simulink model "SRG_Generic_1HpSepExt_13Jan15_mod1"  (Simulink 8.1)
settings: Solver=ode45  StartTime=0.0  StopTime=2.5  FixedStep=Ts  MaxStep=1e-6  MinStep=1e-7  RelTol=1e-5
values from neighbouring files (symbols this model uses):
  Ts = 1e-06    [WorkSpaceBackup1.mat]
undefined symbols (not defined in the file or in its folder): DiscIntNeverNeededParam, find_system
libraries: powerlib x29, simulink x2, powerlib_extras x2, dspsigops x1, DRlib x1
settings Model: Creator=Rahul  LastModifiedBy=USER
settings DataIOCC: SignalLoggingName=signout
settings OptimizationCC: InitFltsAndDblsToZero=on
settings DebuggingCC: CheckExecutionContextPreStartOutputMsg=on  CheckExecutionContextRuntimeOutputMsg=on  SolverPrmCheckMsg=none  MultiTaskDSMMsg=warning  MultiTaskCondExecSysMsg=none
settings HardwareCC: TargetHWDeviceType=32-bit Generic

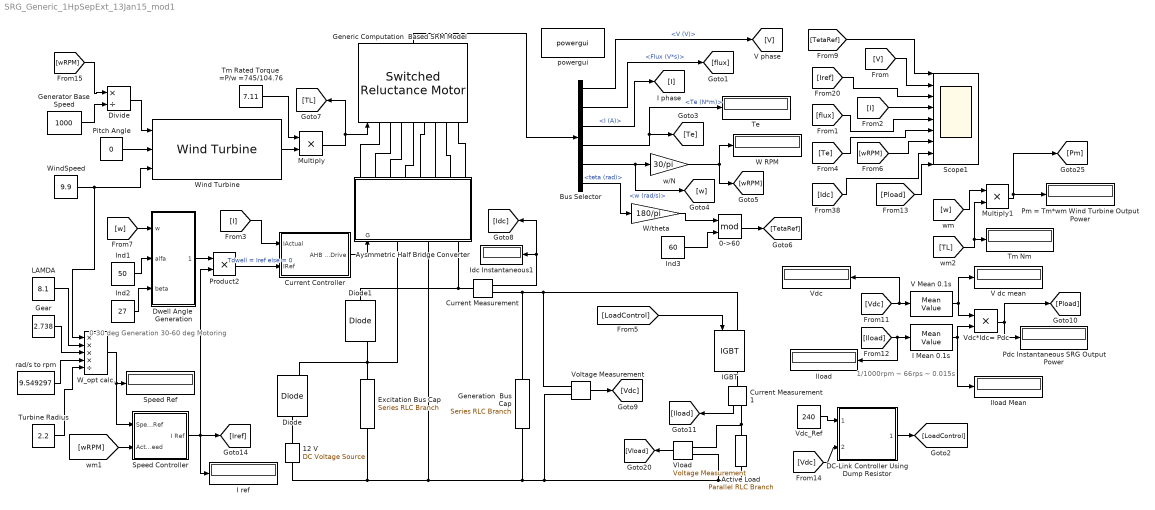
== system SRG_Generic_1HpSepExt_13Jan15_mod1 ==
  note: 1/1000rpm ~ 66rps ~ 0.015s
  note: 0-30 deg Generation
      | 30-60 deg Motoring
  0->60 : Math  Operator=mod  SampleTime=Ts  SaturateOnIntegerOverflow=on
  12 V : powerlib/Electrical Sources/DC Voltage Source  Amplitude=12  Measurements=None
  Active Load : powerlib/Elements/Parallel RLC Branch  LConnTagsString=a  RConnTagsString=__new0  BranchType=R  Resistance=1  Inductance=1e-3  SetiL0=off  InitialCurrent=0  Capacitance=1e-6  Setx0=off  InitialVoltage=0  Measurements=None
  Aysmmetric Half Bridge Converter : Subsystem  LoadFcn=find_system(gcs,'FollowLinks', 'on', 'LookUnderMasks', 'all');
  Bus Selector : BusSelector  OutputSignals=V (V),Flux (V*s),I (A),Te (N*m),w (rad/s),teta (rad)
  Current Controller : Subsystem
  Current Measurement : powerlib/Measurements/Current Measurement  PhasorSimulation=off  OutputType=Complex  PSBequivalent=0
  Current Measurement1 : powerlib/Measurements/Current Measurement  PhasorSimulation=off  OutputType=Complex  PSBequivalent=0
  "DC-Link Controller Using Dump Resistor " : Subsystem
  Diode : powerlib/Power Electronics/Diode  Ron=0.001  Lon=0  Vf=0.8  IC=0  UseSnubber=off  Rs=10e6  Cs=inf  Measurements=on
  Diode1 : powerlib/Power Electronics/Diode  Ron=0.001  Lon=0  Vf=0.8  IC=0  UseSnubber=off  Rs=10e6  Cs=inf  Measurements=on
  Divide : Product  Inputs=*/
  Dwell Angle  Generation : Subsystem
  Excitation Bus Cap : powerlib/Elements/Series RLC Branch  LConnTagsString=__new0  RConnTagsString=__new0  BranchType=RC  Resistance=0.001  Inductance=1e-3  SetiL0=off  InitialCurrent=0  Capacitance=3000e-6  Setx0=on  InitialVoltage=1  Measurements=None
  Gear : Constant  Value=2.738
  Generation  Bus Cap : powerlib/Elements/Series RLC Branch  LConnTagsString=__new0  RConnTagsString=__new0  BranchType=RC  Resistance=0.001  Inductance=1e-3  SetiL0=off  InitialCurrent=0  Capacitance=3000e-6  Setx0=on  InitialVoltage=1  Measurements=None
  Generator Base Speed : Constant  Value=1000
  "Generic Computation  Based SRM Model  " : powerlib/Machines/Switched Reluctance Motor  MachineType=8/6  MachineModel=Generic model  StatorResistance=0.013  PlotCurves=off  Inertia=0.004  Friction=0  InitialSpeed=[97 0]  Lq=0.008  Ld=0.32  Lsat=0.0005  MaximumCurrent=6  MaximumFluxLinkage=0.4  MagnetisationCharacteristic='srm64_60kw.mat'  RotorAngleVector=[0 10 20 30 40 45]  StatorCurrentVector=0:25:450  TsPowergui=0  TsBlock=-1
  I Mean 0.1s : powerlib_extras/Measurements/Mean Value  Period=0.015
  I ref : Display
  IGBT : powerlib/Power Electronics/IGBT  Ron=0.001  Lon=0  Vf=1  Tf=1e-6  Tt=2e-6  IC=0  Rs=1e5  Cs=inf  Measurements=on
  Idc Instantaneous1 : Display
  "Iload " : Display
  Iload Mean : Display
  Ind1 : Constant  Value=50
  Ind2 : Constant  Value=27
  Ind3 : Constant  Value=60
  LAMDA : Constant  Value=8.1
  Multiply : Product  Inputs=**
  Multiply1 : Product  Inputs=**
  Pdc Instantaneous SRG Output Power : Display
  Pitch Angle : Constant  Value=0
  Pm = Tm*wm Wind Turbine Output Power : Display
  Product2 : Product  RndMeth=Zero
  Scope1 : Scope  NumInputPorts=9
      settings: TimeRange=0.1400000000000001  YMin=0~-300~0~-2~-0.1~-10~900~-250~0  YMax=100~300~12~10~0.5~5~1500~250~800  SaveName=ScopeData2  MaxDataPoints=100000
  Speed Controller : Subsystem
  Speed Ref : Display
  Te : Display
  Tm Nm : Display
  Tm Rated Torque =P/w =745/104.76 : Constant  Value=7.11
  Turbine Radius : Constant  Value=2.2
  V Mean 0.1s : powerlib_extras/Measurements/Mean Value  Period=0.015
  V dc mean : Display
  "Vdc " : Display
  Vdc*Idc= Pdc : Product
  Vdc_Ref : Constant  Value=240
  Vload : powerlib/Measurements/Voltage Measurement  PhasorSimulation=off  OutputType=Complex  PSBequivalent=0
  Voltage Measurement : powerlib/Measurements/Voltage Measurement  PhasorSimulation=off  OutputType=Complex  PSBequivalent=0
  W RPM : Display
  W/theta : Gain  Gain=180/pi
  W_opt calc. : Product  Inputs=****/
  Wind Turbine : DRlib/Wind Generation/Wind Turbine  Pnom=1e3  Pelec_base=1e3/0.9  wind_base=12.5  P_wind_base=1  speed_nom=1.2  pitch_angle=0  DisplayTurbChar=off  c1_c6="[0.51763          116          0.4            5           21     0.006795]"  cp_nom=0.48  lambda_nom=8.1
  WindSpeed : Constant  Value=9.9
  powergui : powerlib/powergui  Priority=1  SimulationMode=Discrete  SolverType=Tustin  SampleTime=Ts  frequency=60  SPID=off  DisableSnubberDevices=off  DisableRonSwitches=off  DisableVfSwitches=off  SwTol=0  Interpol=off  DisplayEquations=off  frequencyindice=0  Pbase=100e6  ErrMax=1e-4  Iterations=50  UnitsV=kV  UnitsW=MW  FunctionMessages=off  echomessages=off  HookPort=off  EnableUseOfTLC=off  x0status=blocks  RestoreLinks=warning  ResistiveCurrentMeasurement=off  Frange=[0:2:500]  Ylog=off  Xlog=on  ShowGrid=off  save=off  variable=ZData  ZoomFFT=off  StartTime=0.0  cycles=1  DisplayStyle=1  fundamental=60  FreqAxis=off  MaxFrequency=1000  frequencyindicesteady=1  RmsSteady=1  display=off  Ts=0  methode=off
  rad/s to rpm : Constant  Value=9.549297
  w/N : Gain  Gain=30/pi
  wires:
  "Generic Computation  Based SRM Model  "/1 -> Bus Selector/1
  Bus Selector/6 -> W/theta/1  "<teta (rad)>"
  w/N/1 -> [wRPM], W RPM/1
  Ind3/1 -> 0->60/2
  W/theta/1 -> 0->60/1
  Bus Selector/1 -> [V]  "<V (V)>"
  Bus Selector/2 -> [flux]  "<Flux (V*s)>"
  Bus Selector/3 -> [I]  "<I (A)>"
  Bus Selector/4 -> [Te], Te/1  "<Te (N*m)>"
  Bus Selector/5 -> w/N/1, [w]  "<w (rad/s)>"
  0->60/1 -> [TetaRef]
  Voltage Measurement/1 -> [Vdc]
  Current Measurement/1 -> Idc Instantaneous1/1, [Idc]
  [Iload] -> "Iload "/1, I Mean 0.1s/1
  Vdc*Idc= Pdc/1 -> Pdc Instantaneous SRG Output Power/1, [Pload]
  Current Measurement1/1 -> [Iload]
  [w] -> Multiply1/1
  Multiply1/1 -> [Pm], Pm = Tm*wm Wind Turbine Output Power/1
  [Vdc] -> "Vdc "/1, V Mean 0.1s/1
  I Mean 0.1s/1 -> Iload Mean/1, Vdc*Idc= Pdc/2
  Vload/1 -> [Vload]
  V Mean 0.1s/1 -> V dc mean/1, Vdc*Idc= Pdc/1
  Ind1/1 -> Dwell Angle  Generation/2(alfa)
  Ind2/1 -> Dwell Angle  Generation/3(beta)
  [w] -> Dwell Angle  Generation/1(w)
  [TetaRef] -> Scope1/1
  [V] -> Scope1/2
  [Iref] -> Scope1/3
  [I] -> Scope1/4
  [Pload] -> Scope1/9
  [Idc] -> Scope1/8
  [wRPM] -> Scope1/7
  [Te] -> Scope1/6
  [flux] -> Scope1/5
  [LoadControl] -> IGBT/1
  Vdc_Ref/1 -> "DC-Link Controller Using Dump Resistor "/1(Ref Gen Bus V)
  [Vdc] -> "DC-Link Controller Using Dump Resistor "/2(Actual Gen Bus V)
  "DC-Link Controller Using Dump Resistor "/1(" Load Gate") -> [LoadControl]
  Speed Controller/1(I Ref) -> I ref/1, [Iref], Product2/2
  [wRPM] -> Speed Controller/2(ActualSpeed)
  Product2/1 -> Current Controller/2(IRef)  "Tdwell = Iref else = 0"
  [I] -> Current Controller/1(IActual)
  Current Controller/1(AHB GateDrive) -> Aysmmetric Half Bridge Converter/1(G)
  Dwell Angle  Generation/1(Signal) -> Product2/1
  [wRPM] -> Divide/1
  Generator Base Speed/1 -> Divide/2
  Divide/1 -> Wind Turbine/1
  Pitch Angle/1 -> Wind Turbine/2
  WindSpeed/1 -> W_opt calc./1, Wind Turbine/3
  Multiply/1 -> [TL], "Generic Computation  Based SRM Model  "/1
  Wind Turbine/1 -> Multiply/2
  Tm Rated Torque =P/w =745/104.76/1 -> Multiply/1
  [TL] -> Multiply1/2, Tm Nm/1
  Gear/1 -> W_opt calc./3
  LAMDA/1 -> W_opt calc./2
  Turbine Radius/1 -> W_opt calc./5
  rad/s to rpm/1 -> W_opt calc./4
  W_opt calc./1 -> Speed Ref/1, Speed Controller/1(SpeedRef)
  connections:
  "Generic Computation  Based SRM Model  "/LConn1 -- Aysmmetric Half Bridge Converter/RConn1
  "Generic Computation  Based SRM Model  "/LConn2 -- Aysmmetric Half Bridge Converter/RConn2
  "Generic Computation  Based SRM Model  "/LConn3 -- Aysmmetric Half Bridge Converter/RConn3
  "Generic Computation  Based SRM Model  "/LConn4 -- Aysmmetric Half Bridge Converter/RConn4
  "Generic Computation  Based SRM Model  "/LConn5 -- Aysmmetric Half Bridge Converter/RConn5
  "Generic Computation  Based SRM Model  "/LConn6 -- Aysmmetric Half Bridge Converter/RConn6
  Voltage Measurement/LConn2 -- Active Load/RConn1 -- Vload/LConn2 -- Generation  Bus Cap/RConn1 -- 12 V/LConn1 -- Excitation Bus Cap/RConn1 -- Aysmmetric Half Bridge Converter/LConn2
  Voltage Measurement/LConn1 -- IGBT/LConn1 -- Current Measurement/RConn1 -- Generation  Bus Cap/LConn1
  Diode/LConn1 -- 12 V/RConn1
  Active Load/LConn1 -- Vload/LConn1 -- Current Measurement1/RConn1
  IGBT/RConn1 -- Current Measurement1/LConn1
  Aysmmetric Half Bridge Converter/RConn7 -- "Generic Computation  Based SRM Model  "/LConn7
  Aysmmetric Half Bridge Converter/RConn8 -- "Generic Computation  Based SRM Model  "/LConn8
  Aysmmetric Half Bridge Converter/LConn3 -- Current Measurement/LConn1 -- Diode1/LConn1
  Aysmmetric Half Bridge Converter/LConn1 -- Diode/RConn1 -- Excitation Bus Cap/LConn1 -- Diode1/RConn1

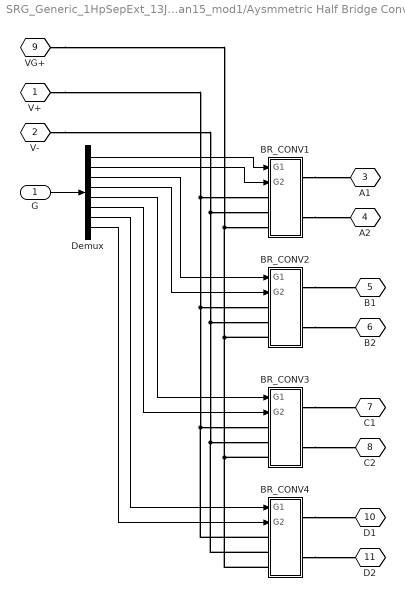
== system SRG_Generic_1HpSepExt_13Jan15_mod1/Aysmmetric Half Bridge Converter ==
  G : Inport
  BR_CONV1 : Subsystem
  BR_CONV2 : Subsystem
  BR_CONV3 : Subsystem
  BR_CONV4 : Subsystem
  Demux : Demux  Outputs=8
  V+ : PMIOPort  Tag=PMCPort  Port=1  Side=Left
  V- : PMIOPort  Tag=PMCPort  Port=2  Side=Left
  A1 : PMIOPort  Tag=PMCPort  Port=3  Side=Right
  A2 : PMIOPort  Tag=PMCPort  Port=4  Side=Right
  B1 : PMIOPort  Tag=PMCPort  Port=5  Side=Right
  B2 : PMIOPort  Tag=PMCPort  Port=6  Side=Right
  C1 : PMIOPort  Tag=PMCPort  Port=7  Side=Right
  C2 : PMIOPort  Tag=PMCPort  Port=8  Side=Right
  VG+ : PMIOPort  Tag=PMCPort  Port=9  Side=Left
  D1 : PMIOPort  Tag=PMCPort  Port=10  Side=Right
  D2 : PMIOPort  Tag=PMCPort  Port=11  Side=Right
  wires:
  G/1 -> Demux/1
  Demux/1 -> BR_CONV1/1(G1)
  Demux/2 -> BR_CONV1/2(G2)
  Demux/3 -> BR_CONV2/1(G1)
  Demux/4 -> BR_CONV2/2(G2)
  Demux/5 -> BR_CONV3/1(G1)
  Demux/6 -> BR_CONV3/2(G2)
  Demux/7 -> BR_CONV4/1(G1)
  Demux/8 -> BR_CONV4/2(G2)
  connections:
  BR_CONV3/RConn2 -- C2/RConn1
  BR_CONV3/RConn1 -- C1/RConn1
  BR_CONV2/RConn2 -- B2/RConn1
  BR_CONV2/RConn1 -- B1/RConn1
  BR_CONV1/RConn2 -- A2/RConn1
  BR_CONV1/RConn1 -- A1/RConn1
  V-/RConn1 -- BR_CONV1/LConn2 -- BR_CONV4/LConn2 -- BR_CONV3/LConn2 -- BR_CONV2/LConn2
  V+/RConn1 -- BR_CONV1/LConn1 -- BR_CONV4/LConn1 -- BR_CONV3/LConn1 -- BR_CONV2/LConn1
  VG+/RConn1 -- BR_CONV1/LConn3 -- BR_CONV4/LConn3 -- BR_CONV3/LConn3 -- BR_CONV2/LConn3
  BR_CONV4/RConn2 -- D2/RConn1
  BR_CONV4/RConn1 -- D1/RConn1

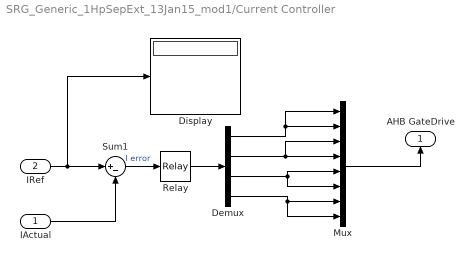
== system SRG_Generic_1HpSepExt_13Jan15_mod1/Current Controller ==
  IActual : Inport
  IRef : Inport  Port=2
  Demux : Demux
  Display : Display
  Mux : Mux  Inputs=8
  Relay : Relay  OnSwitchValue=0.1  OffSwitchValue=-0.1
  Sum1 : Sum  Inputs=|+-
  AHB GateDrive : Outport
  wires:
  IRef/1 -> Display/1, Sum1/1
  Sum1/1 -> Relay/1  "I error"
  IActual/1 -> Sum1/2
  Relay/1 -> Demux/1
  Demux/1 -> Mux/1, Mux/2
  Demux/2 -> Mux/3, Mux/4
  Demux/3 -> Mux/6, Mux/5
  Demux/4 -> Mux/8, Mux/7
  Mux/1 -> AHB GateDrive/1

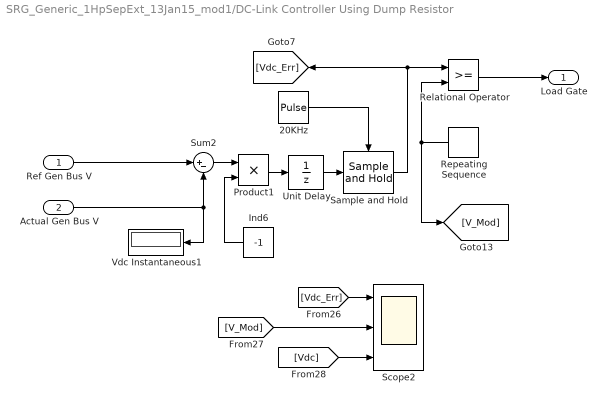
== system SRG_Generic_1HpSepExt_13Jan15_mod1/DC-Link Controller Using Dump Resistor  ==
  Ref Gen Bus V : Inport
  Actual Gen Bus V : Inport  Port=2
  20KHz : DiscretePulseGenerator  PulseType=Time based  Period=0.5e-4  PulseWidth=10
  Ind6 : Constant  Value=-1
  Product1 : Product
  Relational Operator : RelationalOperator  OutDataTypeStr=boolean
  Repeating Sequence : simulink/Sources/Repeating Sequence  rep_seq_t=[0 0.25e-4 0.5e-4]  rep_seq_y=[0 1 0]
  Sample and Hold : dspsigops/Sample and Hold  trig=Rising edge  initCond=0  latchinput=off
  Scope2 : Scope  NumInputPorts=3
      settings: TimeRange=0.1400000000000001  YMin=-5~-2~0  YMax=5~2~300  MaxDataPoints=100000
  Sum2 : Sum  Inputs=|+-
  Unit Delay : UnitDelay  SampleTime=-1
  Vdc Instantaneous1 : Display
  " Load Gate" : Outport
  wires:
  Ref Gen Bus V/1 -> Sum2/1
  Actual Gen Bus V/1 -> Sum2/2, Vdc Instantaneous1/1
  [V_Mod] -> Scope2/2
  [Vdc] -> Scope2/3
  20KHz/1 -> Sample and Hold/Trigger
  Repeating Sequence/1 -> Relational Operator/2, [V_Mod]
  [Vdc_Err] -> Scope2/1
  Ind6/1 -> Product1/2
  Product1/1 -> Unit Delay/1
  Unit Delay/1 -> Sample and Hold/1
  Sample and Hold/1 -> Relational Operator/1, [Vdc_Err]
  Sum2/1 -> Product1/1
  Relational Operator/1 -> " Load Gate"/1

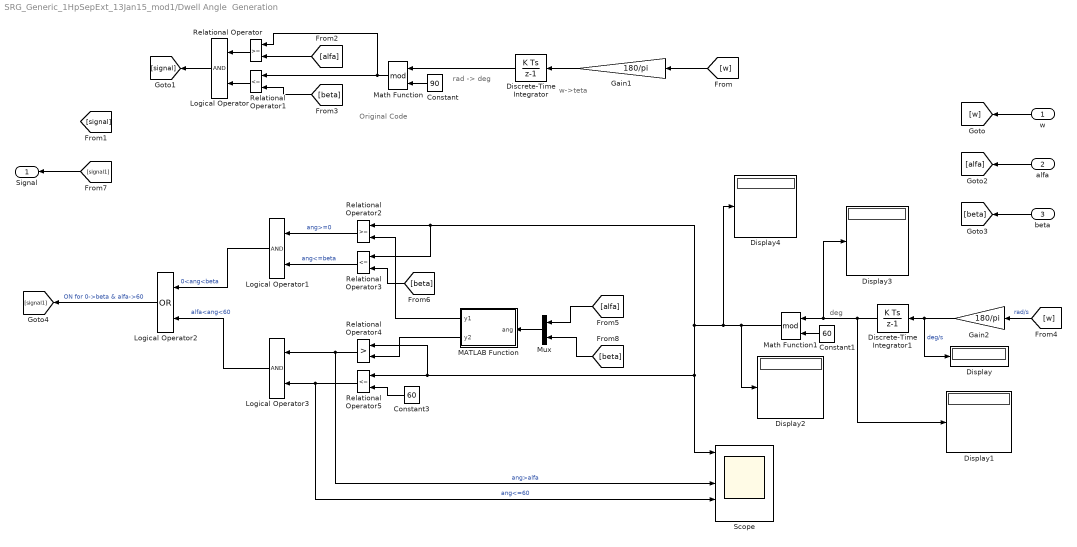
== system SRG_Generic_1HpSepExt_13Jan15_mod1/Dwell Angle  Generation ==
  note: Original Code
  note: rad -> deg
  note: w->teta
  note: deg
  w : Inport
  alfa : Inport  Port=2
  beta : Inport  Port=3
  Constant : Constant  Value=90
  Constant1 : Constant  Value=60
  Constant3 : Constant  Value=60
  Discrete-Time Integrator : DiscreteIntegrator  InitialCondition=[0 -30 -60]  SampleTime=Ts  ICPrevOutput=DiscIntNeverNeededParam  ICPrevScaledInput=DiscIntNeverNeededParam
  Discrete-Time Integrator1 : DiscreteIntegrator  InitialCondition=[0 -15 -30 -45]  SampleTime=Ts  ICPrevOutput=DiscIntNeverNeededParam  ICPrevScaledInput=DiscIntNeverNeededParam
  Display{,1..4} (5 alike) : Display
  Gain1 : Gain  Gain=180/pi  SaturateOnIntegerOverflow=on  OutDataTypeStr=Inherit: Same as input  ParamDataTypeStr=Inherit: Same as input
  Gain2 : Gain  Gain=180/pi  SaturateOnIntegerOverflow=on  OutDataTypeStr=Inherit: Same as input  ParamDataTypeStr=Inherit: Same as input
  Logical Operator : Logic  AllPortsSameDT=off
  Logical Operator1 : Logic  AllPortsSameDT=off
  Logical Operator2 : Logic  Operator=OR  AllPortsSameDT=off
  Logical Operator3 : Logic  AllPortsSameDT=off
  MATLAB Function : MATLAB Function  TreatAsAtomicUnit=on
  Math Function : Math  Operator=mod  SaturateOnIntegerOverflow=on
  Math Function1 : Math  Operator=mod  SaturateOnIntegerOverflow=on
  Mux : Mux  Inputs=2
  Relational Operator : RelationalOperator
  Relational Operator1 : RelationalOperator  Operator=<=
  Relational Operator2 : RelationalOperator
  Relational Operator3 : RelationalOperator  Operator=<=
  Relational Operator4 : RelationalOperator  Operator=>
  Relational Operator5 : RelationalOperator  Operator=<=
  Scope : Scope  NumInputPorts=5
      settings: YMin=-5~-5~-5~-5~-5  YMax=5~5~5~5~5
  Signal : Outport
  wires:
  Math Function/1 -> Relational Operator/1, Relational Operator1/1
  Relational Operator1/1 -> Logical Operator/2
  beta/1 -> [beta]
  alfa/1 -> [alfa]
  Relational Operator/1 -> Logical Operator/1
  Constant/1 -> Math Function/2
  Logical Operator/1 -> [signal]
  Discrete-Time Integrator/1 -> Math Function/1
  Gain1/1 -> Discrete-Time Integrator/1
  w/1 -> [w]
  [w] -> Gain2/1  "rad/s"
  Math Function1/1 -> Display2/1, Relational Operator3/1, Relational Operator2/1, Scope/1, Relational Operator4/1, Relational Operator5/1, Display4/1
  Gain2/1 -> Display/1, Discrete-Time Integrator1/1  "deg/s"
  [beta] -> Relational Operator3/2
  Relational Operator2/1 -> Logical Operator1/1  "ang>=0"
  Constant1/1 -> Math Function1/2
  Discrete-Time Integrator1/1 -> Display1/1, Math Function1/1, Display3/1
  Relational Operator3/1 -> Logical Operator1/2  "ang<=beta"
  Logical Operator1/1 -> Logical Operator2/1  "0<ang<beta"
  Logical Operator3/1 -> Logical Operator2/2  "alfa<ang<60"
  Logical Operator2/1 -> [signal1]  "ON for 0->beta & alfa->60"
  Constant3/1 -> Relational Operator5/2
  Relational Operator4/1 -> Scope/3, Logical Operator3/1  "ang>alfa"
  Relational Operator5/1 -> Scope/4, Logical Operator3/2  "ang<=60"
  MATLAB Function/1(y1) -> Relational Operator2/2
  Mux/1 -> MATLAB Function/1(ang)
  [alfa] -> Mux/1
  [w] -> Gain1/1
  [alfa] -> Relational Operator/2
  [beta] -> Relational Operator1/2
  [signal1] -> Signal/1
  [beta] -> Mux/2
  MATLAB Function/2(y2) -> Relational Operator4/2

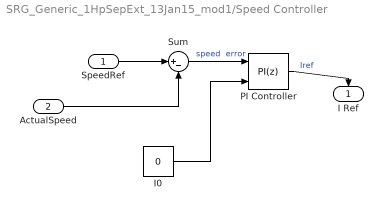
== system SRG_Generic_1HpSepExt_13Jan15_mod1/Speed Controller ==
  SpeedRef : Inport
  ActualSpeed : Inport  Port=2
  I0 : Constant  Value=0
  PI Controller : simulink/Continuous/PID Controller  Controller=PI  TimeDomain=Discrete-time  SampleTime=Ts  IntegratorMethod=Trapezoidal  FilterMethod=Forward Euler  Form=Parallel  P=-1.5  I=0.1  D=0  N=100  InitialConditionSource=external  InitialConditionForIntegrator=0  InitialConditionForFilter=0  ExternalReset=none  ZeroCross=off  LimitOutput=on  UpperSaturationLimit=10  LowerSaturationLimit=0  LinearizeAsGain=off  AntiWindupMode=clamping  Kb=1  TrackingMode=off  Kt=1  PParamMin=[]  PParamMax=[]  IParamMin=[]  IParamMax=[]  DParamMin=[]  DParamMax=[]  NParamMin=[]  NParamMax=[]  KbParamMin=[]  KbParamMax=[]  KtParamMin=[]  KtParamMax=[]  POutMin=[]  POutMax=[]  IOutMin=[]  IOutMax=[]  DOutMin=[]  DOutMax=[]  NOutMin=[]  NOutMax=[]  KbOutMin=[]  KbOutMax=[]  KtOutMin=[]  KtOutMax=[]  IntegratorOutMin=[]  IntegratorOutMax=[]  FilterOutMin=[]  FilterOutMax=[]  SumOutMin=[]  SumOutMax=[]  SumI1OutMin=[]  SumI1OutMax=[]  SumI2OutMin=[]  SumI2OutMax=[]  SumI3OutMin=[]  SumI3OutMax=[]  SumDOutMin=[]  SumDOutMax=[]  SaturationOutMin=[]  SaturationOutMax=[]  IntegratorContinuousStateAttributes=''  IntegratorStateMustResolveToSignalObject=off  IntegratorRTWStateStorageClass=Auto  FilterContinuousStateAttributes=''  FilterStateMustResolveToSignalObject=off  FilterRTWStateStorageClass=Auto
  Sum : Sum  Inputs=|+-
  I Ref : Outport
  wires:
  ActualSpeed/1 -> Sum/2
  Sum/1 -> PI Controller/1  "speed  error"
  PI Controller/1 -> I Ref/1  "Iref"
  SpeedRef/1 -> Sum/1
  I0/1 -> PI Controller/2

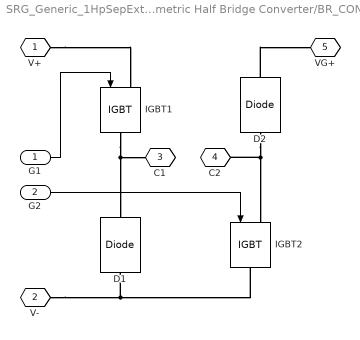
== system SRG_Generic_1HpSepExt_13Jan15_mod1/Aysmmetric Half Bridge Converter/BR_CONV1 ==
  G1 : Inport
  G2 : Inport  Port=2
  D1 : powerlib/Power Electronics/Diode  Ron=1e-3  Lon=0  Vf=0.8  IC=0  UseSnubber=off  Rs=10000  Cs=inf  Measurements=off
  D2 : powerlib/Power Electronics/Diode  Ron=1e-3  Lon=0  Vf=0.8  IC=0  UseSnubber=off  Rs=10000  Cs=inf  Measurements=off
  IGBT1 : powerlib/Power Electronics/IGBT  Ron=1e-3  Lon=0  Vf=1  Tf=0  Tt=0  IC=0  Rs=2000  Cs=0.1e-6  Measurements=off
  IGBT2 : powerlib/Power Electronics/IGBT  Ron=1e-3  Lon=0  Vf=1  Tf=0  Tt=0  IC=0  Rs=2000  Cs=0.1e-6  Measurements=off
  V+ : PMIOPort  Tag=PMCPort  Port=1  Side=Left
  V- : PMIOPort  Tag=PMCPort  Port=2  Side=Left
  C1 : PMIOPort  Tag=PMCPort  Port=3  Side=Right
  C2 : PMIOPort  Tag=PMCPort  Port=4  Side=Right
  VG+ : PMIOPort  Tag=PMCPort  Port=5  Side=Left
  wires:
  G1/1 -> IGBT1/1
  G2/1 -> IGBT2/1
  connections:
  D1/LConn1 -- V-/RConn1 -- IGBT2/RConn1
  D2/LConn1 -- IGBT2/LConn1 -- C2/RConn1
  IGBT1/RConn1 -- D1/RConn1 -- C1/RConn1
  V+/RConn1 -- IGBT1/LConn1
  D2/RConn1 -- VG+/RConn1

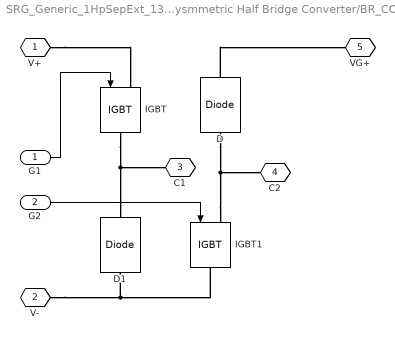
== system SRG_Generic_1HpSepExt_13Jan15_mod1/Aysmmetric Half Bridge Converter/BR_CONV2 ==
  G1 : Inport
  G2 : Inport  Port=2
  D : powerlib/Power Electronics/Diode  Ron=1e-3  Lon=0  Vf=0.8  IC=0  UseSnubber=off  Rs=10000  Cs=inf  Measurements=off
  D1 : powerlib/Power Electronics/Diode  Ron=1e-3  Lon=0  Vf=0.8  IC=0  UseSnubber=off  Rs=10000  Cs=inf  Measurements=off
  IGBT : powerlib/Power Electronics/IGBT  Ron=1e-3  Lon=0  Vf=1  Tf=0  Tt=0  IC=0  Rs=2000  Cs=0.1e-6  Measurements=off
  IGBT1 : powerlib/Power Electronics/IGBT  Ron=1e-3  Lon=0  Vf=1  Tf=0  Tt=0  IC=0  Rs=2000  Cs=0.1e-6  Measurements=off
  V+ : PMIOPort  Tag=PMCPort  Port=1  Side=Left
  V- : PMIOPort  Tag=PMCPort  Port=2  Side=Left
  C1 : PMIOPort  Tag=PMCPort  Port=3  Side=Right
  C2 : PMIOPort  Tag=PMCPort  Port=4  Side=Right
  VG+ : PMIOPort  Tag=PMCPort  Port=5  Side=Left
  wires:
  G1/1 -> IGBT/1
  G2/1 -> IGBT1/1
  connections:
  D1/LConn1 -- V-/RConn1 -- IGBT1/RConn1
  IGBT1/LConn1 -- D/LConn1 -- C2/RConn1
  D1/RConn1 -- IGBT/RConn1 -- C1/RConn1
  V+/RConn1 -- IGBT/LConn1
  D/RConn1 -- VG+/RConn1

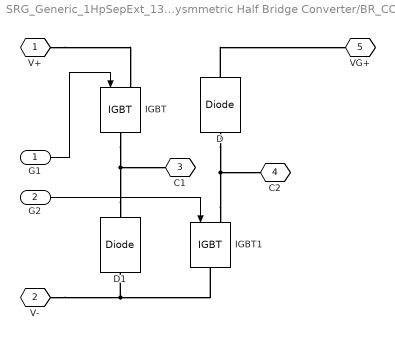
== system SRG_Generic_1HpSepExt_13Jan15_mod1/Aysmmetric Half Bridge Converter/BR_CONV3 ==
  G1 : Inport
  G2 : Inport  Port=2
  D : powerlib/Power Electronics/Diode  Ron=1e-3  Lon=0  Vf=0.8  IC=0  UseSnubber=off  Rs=10000  Cs=inf  Measurements=off
  D1 : powerlib/Power Electronics/Diode  Ron=1e-3  Lon=0  Vf=0.8  IC=0  UseSnubber=off  Rs=10000  Cs=inf  Measurements=off
  IGBT : powerlib/Power Electronics/IGBT  Ron=1e-3  Lon=0  Vf=1  Tf=0  Tt=0  IC=0  Rs=2000  Cs=0.1e-6  Measurements=off
  IGBT1 : powerlib/Power Electronics/IGBT  Ron=1e-3  Lon=0  Vf=1  Tf=0  Tt=0  IC=0  Rs=2000  Cs=0.1e-6  Measurements=off
  V+ : PMIOPort  Tag=PMCPort  Port=1  Side=Left
  V- : PMIOPort  Tag=PMCPort  Port=2  Side=Left
  C1 : PMIOPort  Tag=PMCPort  Port=3  Side=Right
  C2 : PMIOPort  Tag=PMCPort  Port=4  Side=Right
  VG+ : PMIOPort  Tag=PMCPort  Port=5  Side=Left
  wires:
  G1/1 -> IGBT/1
  G2/1 -> IGBT1/1
  connections:
  D1/LConn1 -- V-/RConn1 -- IGBT1/RConn1
  IGBT1/LConn1 -- D/LConn1 -- C2/RConn1
  D1/RConn1 -- IGBT/RConn1 -- C1/RConn1
  V+/RConn1 -- IGBT/LConn1
  D/RConn1 -- VG+/RConn1

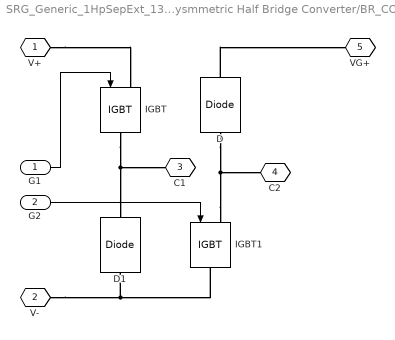
== system SRG_Generic_1HpSepExt_13Jan15_mod1/Aysmmetric Half Bridge Converter/BR_CONV4 ==
  G1 : Inport
  G2 : Inport  Port=2
  D : powerlib/Power Electronics/Diode  Ron=1e-3  Lon=0  Vf=0.8  IC=0  UseSnubber=off  Rs=10000  Cs=inf  Measurements=off
  D1 : powerlib/Power Electronics/Diode  Ron=1e-3  Lon=0  Vf=0.8  IC=0  UseSnubber=off  Rs=10000  Cs=inf  Measurements=off
  IGBT : powerlib/Power Electronics/IGBT  Ron=1e-3  Lon=0  Vf=1  Tf=0  Tt=0  IC=0  Rs=2000  Cs=0.1e-6  Measurements=off
  IGBT1 : powerlib/Power Electronics/IGBT  Ron=1e-3  Lon=0  Vf=1  Tf=0  Tt=0  IC=0  Rs=2000  Cs=0.1e-6  Measurements=off
  V+ : PMIOPort  Tag=PMCPort  Port=1  Side=Left
  V- : PMIOPort  Tag=PMCPort  Port=2  Side=Left
  C1 : PMIOPort  Tag=PMCPort  Port=3  Side=Right
  C2 : PMIOPort  Tag=PMCPort  Port=4  Side=Right
  VG+ : PMIOPort  Tag=PMCPort  Port=5  Side=Left
  wires:
  G1/1 -> IGBT/1
  G2/1 -> IGBT1/1
  connections:
  D1/LConn1 -- V-/RConn1 -- IGBT1/RConn1
  IGBT1/LConn1 -- D/LConn1 -- C2/RConn1
  D1/RConn1 -- IGBT/RConn1 -- C1/RConn1
  V+/RConn1 -- IGBT/LConn1
  D/RConn1 -- VG+/RConn1

== matlab function Dwell Angle Generation/MATLAB Function ==
  data: ang input double; y1 output double; y2 output double
function [y1,y2] = fcn(ang)
%#codegen
alfa=ang(1);
beta=ang(2);
y1=0;
if alfa>beta
    y1=0;
    y2=alfa;
else
    y1=alfa;
    y2=60;   
end
end
